simulink model "servo2"  (R2019a)
settings: Solver=VariableStepAuto  StartTime=0.0  StopTime=18.0  RelTol=1e-3
values from neighbouring files (symbols this model uses):
  A = [0 0 0 0 -23.1569007544 5 0 0 0 6.5 20.5634609555 -3.6 ... (36 elements, 6x6)]    [ABCD.mat]
  B = [0  0; 0  0; 0  0; 24  11.2; 5.55765618105  -1.77142957481; 40  59.4]    [ABCD.mat]
  C_ = [C(1,:); C(3,:)]    [servoctrl2.m]
  K_ = real(inv(R)*Bbar'*P)    [servoctrl2.m]
  x0 = [0.2 -0.1 0.15 -1 0.8 0]    [ABCD.mat]
  y_sp = [3 -5]    [servoctrl2.m]
settings Model: Creator=0210s  LastModifiedBy=0210s

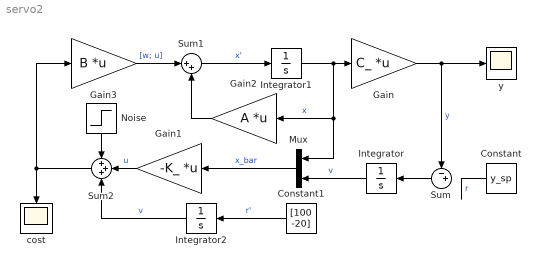
== system servo2 ==
  Constant : Constant  Value=y_sp
  Constant1 : Constant  Value=[100 -20]  VectorParams1D=off
  Gain : Gain  Gain=C_  Multiplication=Matrix(K*u) (u vector)
  Gain1 : Gain  Gain=-K_  Multiplication=Matrix(K*u) (u vector)
  Gain2 : Gain  Gain=A  Multiplication=Matrix(K*u) (u vector)
  Gain3 : Gain  Gain=B  Multiplication=Matrix(K*u) (u vector)
  Integrator : Integrator
  Integrator1 : Integrator  InitialCondition=x0
  Integrator2 : Integrator
  Mux : Mux  Inputs=2
  Noise : Step  Time=10  Before=[0 0]  After=[-1 1]  SampleTime=0  VectorParams1D=off
  Sum : Sum  Inputs=-+|
  Sum1 : Sum  Inputs=|++
  Sum2 : Sum  Inputs=+++
  cost : Scope
  y : Scope
  wires:
  Integrator/1 -> Mux/2  "v"
  Sum/1 -> Integrator/1
  Constant/1 -> ?  "r"
  Gain/1 -> y/1, Sum/1  "y"
  Mux/1 -> Gain1/1  "x_bar"
  Integrator1/1 -> Gain/1, Gain2/1, Mux/1  "x"
  Gain2/1 -> Sum1/2
  Sum1/1 -> Integrator1/1  "x'"
  Gain3/1 -> Sum1/1  "[w; u]"
  Gain1/1 -> Sum2/2  "u"
  Noise/1 -> Sum2/1
  Sum2/1 -> cost/1, Gain3/1
  Constant1/1 -> Integrator2/1  "r'"
  Integrator2/1 -> Sum2/3  "v"
